simulink model "controlador19"  (R2021a)
settings: Solver=ode23t  StartTime=0.0  StopTime=60  MaxStep=1e-3  RelTol=1e-3
values from neighbouring files (symbols this model uses):
  Ac_2 = [AL-BL*Kes-L*CL+L*DL*Kes, BL*Ki - L*DL*Ki ... (first row only)    [modeloMATEMATICOFINAL.m]
  AL = double(subs(A_par))    [modeloMATEMATICOFINAL.m]
  Bc_2 = [zeros(n,r),L ... (first row only)    [modeloMATEMATICOFINAL.m]
  BL = double(subs(B_par))    [modeloMATEMATICOFINAL.m]
  Blo = 8.18575752786119e-06    (= 8.18575752786e-06)    [modeloMATEMATICOFINAL.m]
  Bmo = 2.02156082362446e-07    (= 2.02156082362e-07)    [modeloMATEMATICOFINAL.m]
  Cc_2 = [-Kes, Ki]    [modeloMATEMATICOFINAL.m]
  CL = double(subs(C_par))    [modeloMATEMATICOFINAL.m]
  Dc_2 = zeros(p,2*r)    [modeloMATEMATICOFINAL.m]
  DL = double(subs(D_par))    [modeloMATEMATICOFINAL.m]
  do = 0.06862-0.021    (= 0.04762)    [modeloMATEMATICOFINAL.m]
  GL = sysd.a    [modeloMATEMATICOFINAL.m]
  go = 9.81    [modeloMATEMATICOFINAL.m]
  HL = sysd.b    [modeloMATEMATICOFINAL.m]
  Jlo = 0.00100697016255642    (= 0.00100697016256)    [modeloMATEMATICOFINAL.m]
  Jmo = 2.08549279330578e-07    (= 2.08549279331e-07)    [modeloMATEMATICOFINAL.m]
  Kes = K(:,1:n)    [modeloMATEMATICOFINAL.m]
  Kest = Kt(:,1:n)    [modeloMATEMATICOFINAL.m]
  Ki = -Kt(:,n+1:end)    [modeloMATEMATICOFINAL.m]
  Kio = 0.00119530882984502    (= 0.00119530882985)    [modeloMATEMATICOFINAL.m]
  Kvo = 0.0035694528924319    (= 0.00356945289243)    [modeloMATEMATICOFINAL.m]
  L = place(GL',CL',pol_obv_d)'    [modeloMATEMATICOFINAL.m]
  Lo = 0.667669785204658    (= 0.667669785205)    [modeloMATEMATICOFINAL.m]
  mo = 0.17244    [modeloMATEMATICOFINAL.m]
  no = 120    [modeloMATEMATICOFINAL.m]
  Ro = 5.15610211779038    (= 5.15610211779)    [modeloMATEMATICOFINAL.m]
  sys_d2 = c2d(sys_c2,Tm)    [modeloMATEMATICOFINAL.m]
  Tm = 0.03    [modeloMATEMATICOFINAL.m]
  Vin0 = Ro*X10    (= 0)    [modeloMATEMATICOFINAL.m]
  X10 = 0    [modeloMATEMATICOFINAL.m]
  X20 = 0    [modeloMATEMATICOFINAL.m]
  X30 = 0    [modeloMATEMATICOFINAL.m]
undefined symbols (not defined in the file or in its folder): magnitude
libraries: simulink x8
settings Model: Creator=hubertdelgado  LastModifiedBy=hubertdelgado

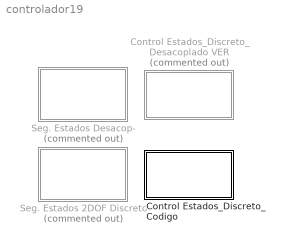
== system controlador19 ==
  Control Estados_Discreto_Codigo : Subsystem
  Control Estados_Discreto_Desacoplado VER : Subsystem  Commented=on
  Seg. Estados 2DOF Discreto : Subsystem  Commented=on
  Seg. Estados Desacop- : Subsystem  Commented=on

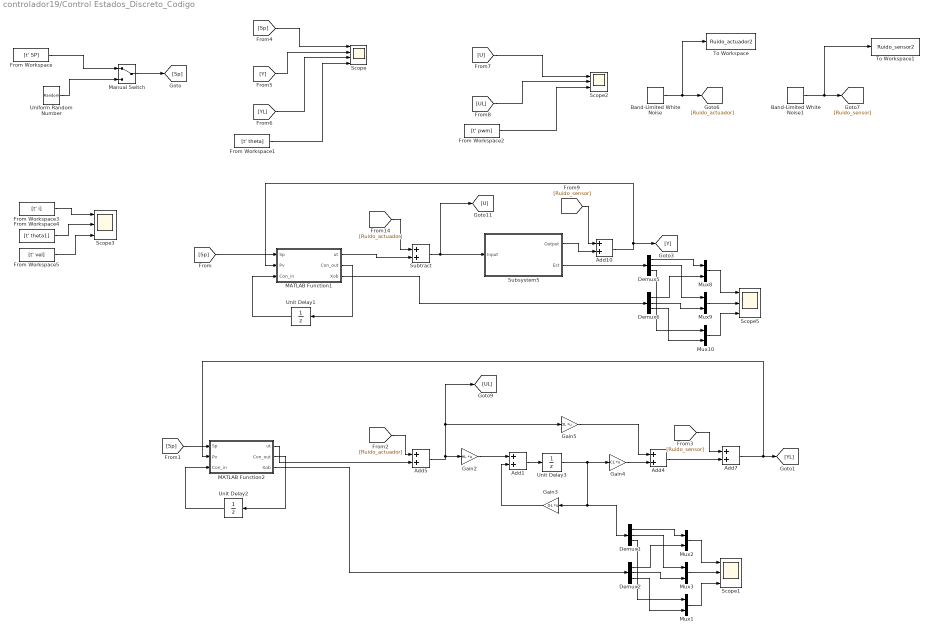
== system controlador19/Control Estados_Discreto_Codigo ==
  Add{1,4..5,7,10} (5 alike) : Sum
  Band-Limited White Noise : simulink/Sources/Band-Limited White Noise  Cov=[1e-8]  Ts=0.001  seed=[23341]
  Band-Limited White Noise1 : simulink/Sources/Band-Limited White Noise  Cov=[1e-8]  Ts=0.001  seed=[23341]
  Demux{1..2,5..6} (4 alike) : Demux  Outputs=3
  From Workspace : FromWorkspace  VariableName=[t' SP]
  From Workspace1 : FromWorkspace  VariableName=[t' theta]
  From Workspace2 : FromWorkspace  VariableName=[t' pwm]
  From Workspace3 : FromWorkspace  VariableName=[t' i]
  From Workspace4 : FromWorkspace  VariableName=[t' theta1]
  From Workspace5 : FromWorkspace  VariableName=[t' vel]
  Gain2 : Gain  Gain=HL  Multiplication=Matrix(K*u)
  Gain3 : Gain  Gain=GL  Multiplication=Matrix(K*u)
  Gain4 : Gain  Gain=CL  Multiplication=Matrix(K*u)
  Gain5 : Gain  Gain=DL  Multiplication=Matrix(K*u)
  MATLAB Function1 : MATLAB Function  TreatAsAtomicUnit=on
  MATLAB Function2 : MATLAB Function  TreatAsAtomicUnit=on
  Manual Switch : ManualSwitch
  Mux{1..3,8..10} (6 alike) : Mux  Inputs=2
  Scope : Scope  NumInputPorts=4
  Scope{1..3,5} (4 alike) : Scope  NumInputPorts=3
  Subsystem5 : Subsystem
  Subtract : Sum
  To Workspace : ToWorkspace  VariableName=Ruido_actuador2  SampleTime=-1
  To Workspace1 : ToWorkspace  VariableName=Ruido_sensor2  SampleTime=-1
  Uniform Random Number : UniformRandomNumber  Minimum=-60*(pi/180)  Maximum=60*(pi/180)  SampleTime=10
  Unit Delay1 : UnitDelay  InitialCondition=zeros(5,1)  SampleTime=Tm  HasFrameUpgradeWarning=on
  Unit Delay2 : UnitDelay  InitialCondition=zeros(5,1)  SampleTime=Tm  HasFrameUpgradeWarning=on
  Unit Delay3 : UnitDelay  SampleTime=Tm  HasFrameUpgradeWarning=on
  wires:
  Add5/1 -> [UL], Gain5/1, Gain2/1
  Add4/1 -> Add7/2
  [Ruido_sensor] -> Add10/1
  [Ruido_actuador] -> Subtract/1
  [Ruido_sensor] -> Add7/1
  Add7/1 -> MATLAB Function2/2(Pv), [YL]
  Gain5/1 -> Add4/1
  Subsystem5/1(Output) -> Add10/2
  MATLAB Function2/1(ut) -> Add5/2
  Subtract/1 -> Subsystem5/1(Input), [U]
  Gain4/1 -> Add4/2
  [Sp] -> MATLAB Function2/1(Sp)
  Band-Limited White Noise/1 -> To Workspace/1, [Ruido_actuador]
  Band-Limited White Noise1/1 -> To Workspace1/1, [Ruido_sensor]
  Gain2/1 -> Add1/1
  Gain3/1 -> Add1/2
  Add1/1 -> Unit Delay3/1
  [Ruido_actuador] -> Add5/1
  MATLAB Function1/2(Con_out) -> Unit Delay1/1
  [Sp] -> MATLAB Function1/1(Sp)
  Unit Delay1/1 -> MATLAB Function1/3(Con_in)
  MATLAB Function1/1(ut) -> Subtract/2
  Add10/1 -> MATLAB Function1/2(Pv), [Y]
  MATLAB Function2/2(Con_out) -> Unit Delay2/1
  Unit Delay2/1 -> MATLAB Function2/3(Con_in)
  Mux8/1 -> Scope5/1
  Mux9/1 -> Scope5/2
  Demux5/3 -> Mux10/1
  Subsystem5/2(Est) -> Demux5/1
  Demux5/1 -> Mux8/1
  Mux10/1 -> Scope5/3
  Demux5/2 -> Mux9/1
  Mux2/1 -> Scope1/1
  Mux3/1 -> Scope1/2
  Demux2/3 -> Mux1/2
  Demux1/3 -> Mux1/1
  Unit Delay3/1 -> Gain4/1, Demux1/1, Gain3/1
  MATLAB Function2/3(Xob) -> Demux2/1
  Demux2/2 -> Mux3/2
  Demux2/1 -> Mux2/2
  Demux1/1 -> Mux2/1
  Mux1/1 -> Scope1/3
  Demux1/2 -> Mux3/1
  From Workspace/1 -> Manual Switch/1
  [Y] -> Scope/2
  From Workspace1/1 -> Scope/4
  Manual Switch/1 -> [Sp]
  [YL] -> Scope/3
  From Workspace2/1 -> Scope2/3
  [UL] -> Scope2/2
  [U] -> Scope2/1
  Uniform Random Number/1 -> Manual Switch/2
  [Sp] -> Scope/1
  From Workspace3/1 -> Scope3/1
  From Workspace4/1 -> Scope3/2
  From Workspace5/1 -> Scope3/3
  MATLAB Function1/3(Xob) -> Demux6/1
  Demux6/1 -> Mux8/2
  Demux6/2 -> Mux9/2
  Demux6/3 -> Mux10/2

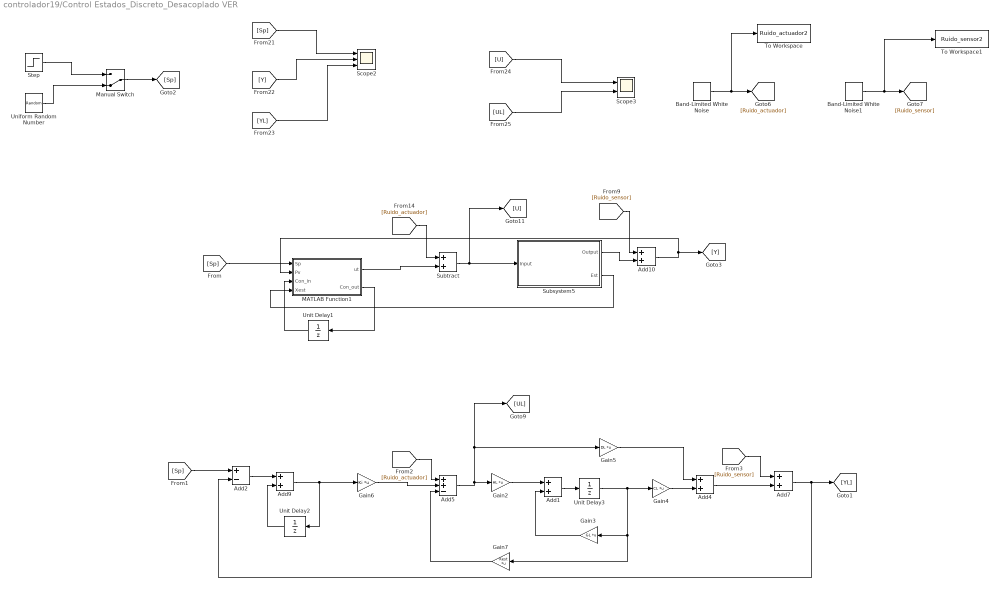
== system controlador19/Control Estados_Discreto_Desacoplado VER ==
  Add{1,4,7,9..10} (5 alike) : Sum
  Add2 : Sum  Inputs=+-
  Add5 : Sum  Inputs=++-
  Band-Limited White Noise : simulink/Sources/Band-Limited White Noise  Cov=[1e-8]  Ts=0.001  seed=[23341]
  Band-Limited White Noise1 : simulink/Sources/Band-Limited White Noise  Cov=[1e-8]  Ts=0.001  seed=[23341]
  Gain2 : Gain  Gain=HL  Multiplication=Matrix(K*u)
  Gain3 : Gain  Gain=GL  Multiplication=Matrix(K*u)
  Gain4 : Gain  Gain=CL  Multiplication=Matrix(K*u)
  Gain5 : Gain  Gain=DL  Multiplication=Matrix(K*u)
  Gain6 : Gain  Gain=Ki  Multiplication=Matrix(K*u)
  Gain7 : Gain  Gain=Kest  Multiplication=Matrix(K*u)
  MATLAB Function1 : MATLAB Function  TreatAsAtomicUnit=on
  Manual Switch : ManualSwitch  CurrentSetting=0
  Scope2 : Scope  NumInputPorts=3
  Scope3 : Scope  NumInputPorts=2
  Step : Step  Time=0  After=30*(pi/180)  SampleTime=0
  Subsystem5 : Subsystem
  Subtract : Sum
  To Workspace : ToWorkspace  VariableName=Ruido_actuador2  SampleTime=-1
  To Workspace1 : ToWorkspace  VariableName=Ruido_sensor2  SampleTime=-1
  Uniform Random Number : UniformRandomNumber  Minimum=-60*(pi/180)  Maximum=60*(pi/180)  SampleTime=10
  Unit Delay1 : UnitDelay  InitialCondition=zeros(2,1)  SampleTime=Tm  HasFrameUpgradeWarning=on
  Unit Delay2 : UnitDelay  SampleTime=Tm  HasFrameUpgradeWarning=on
  Unit Delay3 : UnitDelay  SampleTime=Tm  HasFrameUpgradeWarning=on
  wires:
  [Sp] -> Scope2/1
  Add5/1 -> [UL], Gain5/1, Gain2/1
  Add4/1 -> Add7/2
  [Ruido_sensor] -> Add10/1
  [Ruido_actuador] -> Subtract/1
  [Ruido_sensor] -> Add7/1
  Add7/1 -> Add2/2, [YL]
  Gain5/1 -> Add4/1
  [Y] -> Scope2/2
  Subsystem5/1(Output) -> Add10/2
  [YL] -> Scope2/3
  Subtract/1 -> Subsystem5/1(Input), [U]
  Gain4/1 -> Add4/2
  Band-Limited White Noise/1 -> To Workspace/1, [Ruido_actuador]
  Band-Limited White Noise1/1 -> To Workspace1/1, [Ruido_sensor]
  Manual Switch/1 -> [Sp]
  [UL] -> Scope3/2
  Step/1 -> Manual Switch/1
  [U] -> Scope3/1
  Uniform Random Number/1 -> Manual Switch/2
  Gain2/1 -> Add1/1
  Gain3/1 -> Add1/2
  Add1/1 -> Unit Delay3/1
  [Ruido_actuador] -> Add5/1
  MATLAB Function1/2(Con_out) -> Unit Delay1/1
  [Sp] -> MATLAB Function1/1(Sp)
  Unit Delay1/1 -> MATLAB Function1/3(Con_in)
  MATLAB Function1/1(ut) -> Subtract/2
  Add10/1 -> MATLAB Function1/2(Pv), [Y]
  Unit Delay3/1 -> Gain4/1, Gain7/1, Gain3/1
  Subsystem5/2(Est) -> MATLAB Function1/4(Xest)
  Add9/1 -> Gain6/1, Unit Delay2/1
  Add2/1 -> Add9/1
  Unit Delay2/1 -> Add9/2
  [Sp] -> Add2/1
  Gain6/1 -> Add5/2
  Gain7/1 -> Add5/3

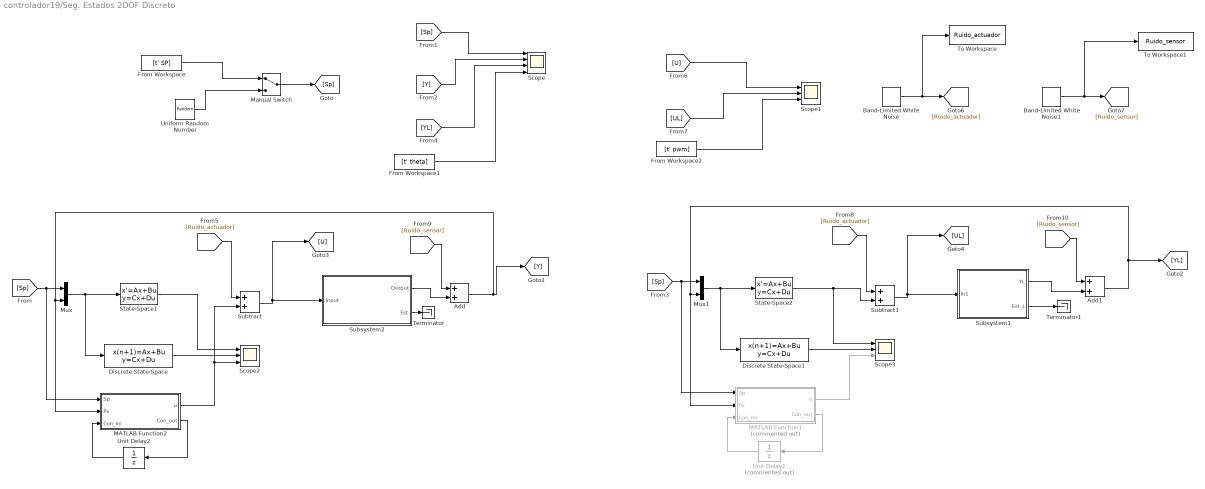
== system controlador19/Seg. Estados 2DOF Discreto ==
  Add : Sum
  Add1 : Sum
  Band-Limited White Noise : simulink/Sources/Band-Limited White Noise  Cov=[1e-8]  Ts=0.001  seed=[23341]
  Band-Limited White Noise1 : simulink/Sources/Band-Limited White Noise  Cov=[1e-8]  Ts=0.001  seed=[23341]
  Discrete State-Space : DiscreteStateSpace  A=sys_d2.a  B=sys_d2.b  C=sys_d2.c  D=sys_d2.d  SampleTime=Tm
  Discrete State-Space1 : DiscreteStateSpace  A=sys_d2.a  B=sys_d2.b  C=sys_d2.c  D=sys_d2.d  SampleTime=Tm
  From Workspace : FromWorkspace  VariableName=[t' SP]
  From Workspace1 : FromWorkspace  VariableName=[t' theta]
  From Workspace2 : FromWorkspace  VariableName=[t' pwm]
  MATLAB Function1 : MATLAB Function  Commented=on  TreatAsAtomicUnit=on
  MATLAB Function2 : MATLAB Function  TreatAsAtomicUnit=on
  Manual Switch : ManualSwitch
  Mux : Mux  Inputs=2
  Mux1 : Mux  Inputs=2
  Scope : Scope  NumInputPorts=4
  Scope1 : Scope  NumInputPorts=3
  Scope2 : Scope  NumInputPorts=3
  Scope3 : Scope  NumInputPorts=3
  State-Space1 : StateSpace  A=Ac_2  B=Bc_2  C=Cc_2  D=Dc_2  InitialCondition=0
  State-Space2 : StateSpace  A=Ac_2  B=Bc_2  C=Cc_2  D=Dc_2  InitialCondition=0
  Subsystem1 : Subsystem
  Subsystem2 : Subsystem
  Subtract : Sum
  Subtract1 : Sum
  Terminator : Terminator
  Terminator1 : Terminator
  To Workspace : ToWorkspace  VariableName=Ruido_actuador  SampleTime=-1
  To Workspace1 : ToWorkspace  VariableName=Ruido_sensor  SampleTime=-1
  Uniform Random Number : UniformRandomNumber  Minimum=-60*(pi/180)  Maximum=60*(pi/180)  SampleTime=10
  Unit Delay1 : UnitDelay  Commented=on  InitialCondition=zeros(8,1)  SampleTime=Tm  HasFrameUpgradeWarning=on
  Unit Delay2 : UnitDelay  InitialCondition=zeros(5,1)  SampleTime=Tm  HasFrameUpgradeWarning=on
  wires:
  [Sp] -> MATLAB Function2/1(Sp), Mux/1
  Band-Limited White Noise/1 -> To Workspace/1, [Ruido_actuador]
  Band-Limited White Noise1/1 -> To Workspace1/1, [Ruido_sensor]
  [UL] -> Scope1/2
  Uniform Random Number/1 -> Manual Switch/2
  [Sp] -> Scope/1
  From Workspace/1 -> Manual Switch/1
  Manual Switch/1 -> [Sp]
  [YL] -> Scope/3
  Subtract/1 -> Subsystem2/1(Input), [U]
  State-Space1/1 -> Scope2/1
  [Ruido_actuador] -> Subtract/1
  Add/1 -> MATLAB Function2/2(Pv), Mux/2, [Y]
  Subsystem2/1(Output) -> Add/2
  [Ruido_sensor] -> Add/1
  Subsystem2/2(Est) -> Terminator/1
  Mux/1 -> Discrete State-Space/1, State-Space1/1
  Discrete State-Space/1 -> Scope2/2
  MATLAB Function2/2(Con_out) -> Unit Delay2/1
  Unit Delay2/1 -> MATLAB Function2/3(Con_ini)
  MATLAB Function2/1(u) -> Subtract/2, Scope2/3
  [Sp] -> MATLAB Function1/1(Sp), Mux1/1
  Subsystem1/2(Est_L) -> Terminator1/1
  MATLAB Function1/1(u) -> Scope3/3
  [Ruido_sensor] -> Add1/1
  Subsystem1/1(YL) -> Add1/2
  Add1/1 -> MATLAB Function1/2(Pv), Mux1/2, [YL]
  Subtract1/1 -> Subsystem1/1(In1), [UL]
  [Ruido_actuador] -> Subtract1/1
  Discrete State-Space1/1 -> Scope3/2
  Unit Delay1/1 -> MATLAB Function1/3(Con_ini)
  Mux1/1 -> Discrete State-Space1/1, State-Space2/1
  State-Space2/1 -> Scope3/1, Subtract1/2
  MATLAB Function1/2(Con_out) -> Unit Delay1/1
  From Workspace1/1 -> Scope/4
  From Workspace2/1 -> Scope1/3
  [Y] -> Scope/2
  [U] -> Scope1/1

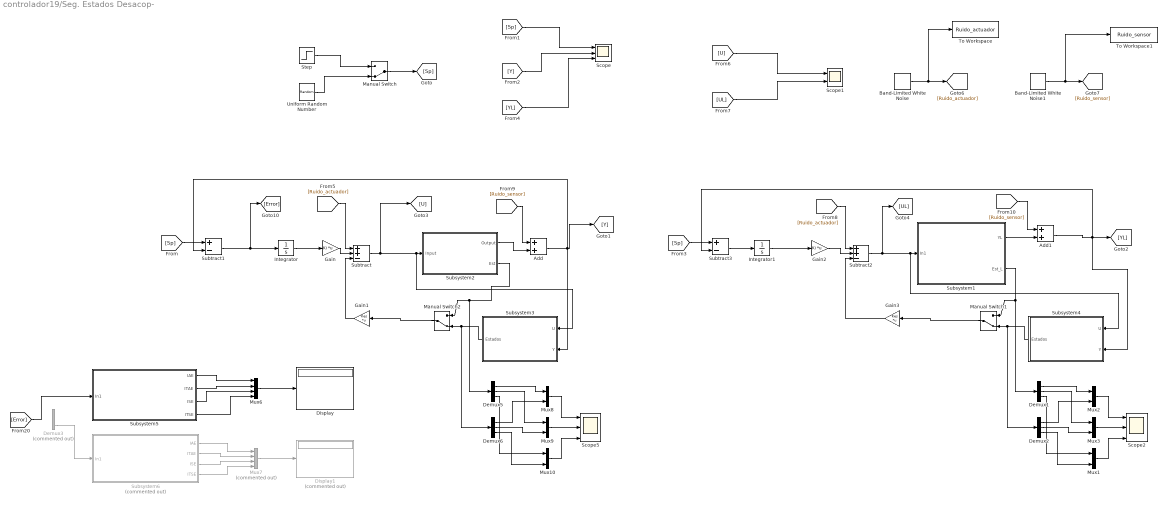
== system controlador19/Seg. Estados Desacop- ==
  Add : Sum
  Add1 : Sum
  Band-Limited White Noise : simulink/Sources/Band-Limited White Noise  Cov=[1e-8]  Ts=0.001  seed=[23341]
  Band-Limited White Noise1 : simulink/Sources/Band-Limited White Noise  Cov=[1e-8]  Ts=0.001  seed=[23341]
  Demux{1..2,5..6} (4 alike) : Demux  Outputs=3
  Demux3 : Demux  Commented=on  Outputs=2
  Display : Display
  Display1 : Display  Commented=on
  Gain : Gain  Gain=Ki  Multiplication=Matrix(K*u)
  Gain1 : Gain  Gain=Kes  Multiplication=Matrix(K*u)
  Gain2 : Gain  Gain=Ki  Multiplication=Matrix(K*u)
  Gain3 : Gain  Gain=Kes  Multiplication=Matrix(K*u)
  Integrator : Integrator
  Integrator1 : Integrator
  Manual Switch : ManualSwitch  CurrentSetting=0
  Manual Switch1 : ManualSwitch  CurrentSetting=0
  Manual Switch2 : ManualSwitch  CurrentSetting=0
  Mux{1..3,8..10} (6 alike) : Mux  Inputs=2
  Mux6 : Mux
  Mux7 : Mux  Commented=on
  Scope : Scope  NumInputPorts=3
  Scope1 : Scope  NumInputPorts=2
  Scope2 : Scope  NumInputPorts=3
  Scope5 : Scope  NumInputPorts=3
  Step : Step  Time=0  After=0  SampleTime=0
  Subsystem1 : Subsystem
  Subsystem2 : Subsystem
  Subsystem3 : Subsystem
  Subsystem4 : Subsystem
  Subsystem5 : Subsystem
  Subsystem6 : Subsystem  Commented=on
  Subtract : Sum  Inputs=++-
  Subtract1 : Sum  Inputs=+-
  Subtract2 : Sum  Inputs=++-
  Subtract3 : Sum  Inputs=+-
  To Workspace : ToWorkspace  VariableName=Ruido_actuador  SampleTime=-1
  To Workspace1 : ToWorkspace  VariableName=Ruido_sensor  SampleTime=-1
  Uniform Random Number : UniformRandomNumber  Minimum=-60*(pi/180)  Maximum=60*(pi/180)  SampleTime=10
  wires:
  [Sp] -> Subtract1/1
  [Sp] -> Subtract3/1
  Integrator/1 -> Gain/1
  Integrator1/1 -> Gain2/1
  Subtract3/1 -> Integrator1/1
  Band-Limited White Noise/1 -> To Workspace/1, [Ruido_actuador]
  Band-Limited White Noise1/1 -> To Workspace1/1, [Ruido_sensor]
  [UL] -> Scope1/2
  Uniform Random Number/1 -> Manual Switch/2
  [Sp] -> Scope/1
  [U] -> Scope1/1
  Step/1 -> Manual Switch/1
  Manual Switch/1 -> [Sp]
  [YL] -> Scope/3
  [Y] -> Scope/2
  Subtract/1 -> Subsystem3/1(U), Subsystem2/1(Input), [U]
  Mux10/1 -> Scope5/3
  Demux6/1 -> Mux8/2
  Demux5/2 -> Mux9/1
  Mux8/1 -> Scope5/1
  Demux6/3 -> Mux10/2
  Demux6/2 -> Mux9/2
  Demux5/3 -> Mux10/1
  Mux9/1 -> Scope5/2
  Subsystem3/1(Estados) -> Demux6/1, Manual Switch2/2
  Subsystem2/2(Est) -> Demux5/1, Manual Switch2/1
  Manual Switch2/1 -> Gain1/1
  Subtract2/1 -> [UL], Subsystem4/1(U), Subsystem1/1(In1)
  Mux1/1 -> Scope2/3
  Demux2/1 -> Mux2/2
  Demux1/2 -> Mux3/1
  Mux2/1 -> Scope2/1
  Demux2/3 -> Mux1/2
  Demux2/2 -> Mux3/2
  Demux1/3 -> Mux1/1
  Mux3/1 -> Scope2/2
  Subsystem4/1(Estados) -> Demux2/1, Manual Switch1/2
  Demux1/1 -> Mux2/1
  Subsystem1/2(Est_L) -> Demux1/1, Manual Switch1/1
  Manual Switch1/1 -> Gain3/1
  Subtract1/1 -> [Error], Integrator/1
  Subsystem5/2(ITAE) -> Mux6/2
  Subsystem5/4(ITSE) -> Mux6/4
  Subsystem5/3(ISE) -> Mux6/3
  Subsystem5/1(IAE) -> Mux6/1
  Mux7/1 -> Display1/1
  Subsystem6/1(IAE) -> Mux7/1
  Subsystem6/4(ITSE) -> Mux7/4
  Mux6/1 -> Display/1
  Demux3/2 -> Subsystem6/1(In1)
  Subsystem6/3(ISE) -> Mux7/3
  Subsystem6/2(ITAE) -> Mux7/2
  [Error] -> Subsystem5/1(In1)
  Gain/1 -> Subtract/2
  Gain1/1 -> Subtract/3
  [Ruido_actuador] -> Subtract/1
  Gain2/1 -> Subtract2/2
  Gain3/1 -> Subtract2/3
  [Ruido_actuador] -> Subtract2/1
  Add/1 -> Subtract1/2, Subsystem3/2(Y), [Y]
  Subsystem2/1(Output) -> Add/2
  [Ruido_sensor] -> Add/1
  Subsystem1/1(YL) -> Add1/2
  Add1/1 -> Subsystem4/2(Y), Subtract3/2, [YL]
  [Ruido_sensor] -> Add1/1
  Demux5/1 -> Mux8/1

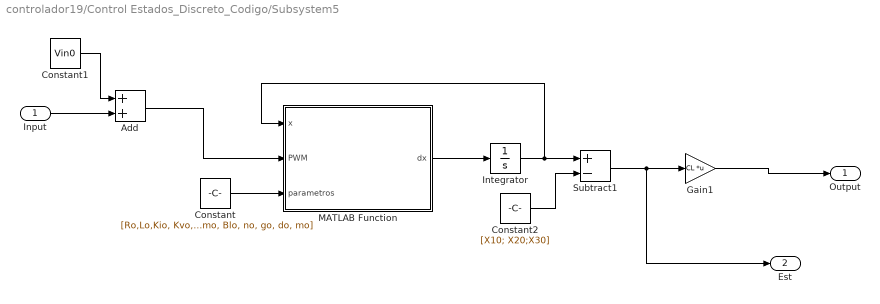
== system controlador19/Control Estados_Discreto_Codigo/Subsystem5 ==
  Input : Inport
  Add : Sum
  Constant : Constant  Value=[Ro,Lo,Kio, Kvo, Jmo, Jlo, Bmo, Blo, no, go, do, mo]
  Constant1 : Constant  Value=Vin0
  Constant2 : Constant  Value=[X10; X20;X30]
  Gain1 : Gain  Gain=CL  Multiplication=Matrix(K*u)
  Integrator : Integrator  InitialCondition=[X10; X20;X30]
  MATLAB Function : MATLAB Function  TreatAsAtomicUnit=on
  Subtract1 : Sum  Inputs=+-
  Output : Outport
  Est : Outport  Port=2
  wires:
  Add/1 -> MATLAB Function/2(PWM)
  Constant2/1 -> Subtract1/2
  Constant1/1 -> Add/1
  Input/1 -> Add/2
  MATLAB Function/1(dx) -> Integrator/1
  Constant/1 -> MATLAB Function/3(parametros)
  Integrator/1 -> Subtract1/1, MATLAB Function/1(x)
  Subtract1/1 -> Est/1, Gain1/1
  Gain1/1 -> Output/1

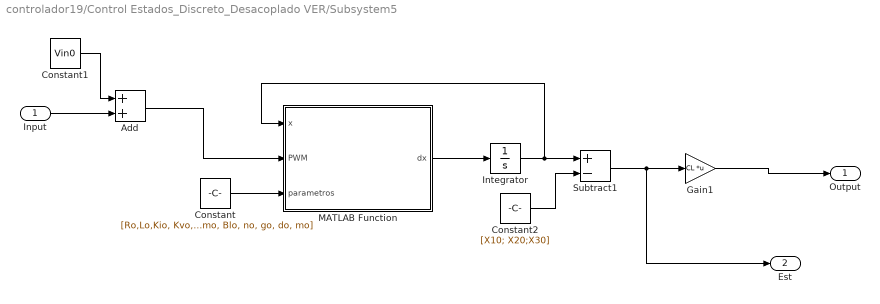
== system controlador19/Control Estados_Discreto_Desacoplado VER/Subsystem5 ==
  Input : Inport
  Add : Sum
  Constant : Constant  Value=[Ro,Lo,Kio, Kvo, Jmo, Jlo, Bmo, Blo, no, go, do, mo]
  Constant1 : Constant  Value=Vin0
  Constant2 : Constant  Value=[X10; X20;X30]
  Gain1 : Gain  Gain=CL  Multiplication=Matrix(K*u)
  Integrator : Integrator  InitialCondition=[X10; X20;X30]
  MATLAB Function : MATLAB Function  TreatAsAtomicUnit=on
  Subtract1 : Sum  Inputs=+-
  Output : Outport
  Est : Outport  Port=2
  wires:
  Add/1 -> MATLAB Function/2(PWM)
  Constant2/1 -> Subtract1/2
  Constant1/1 -> Add/1
  Input/1 -> Add/2
  MATLAB Function/1(dx) -> Integrator/1
  Constant/1 -> MATLAB Function/3(parametros)
  Integrator/1 -> Subtract1/1, MATLAB Function/1(x)
  Subtract1/1 -> Est/1, Gain1/1
  Gain1/1 -> Output/1

== system controlador19/Seg. Estados 2DOF Discreto/Subsystem1 ==
  In1 : Inport
  Add : Sum
  Add1 : Sum
  Gain : Gain  Gain=CL  Multiplication=Matrix(K*u)
  Gain1 : Gain  Gain=AL  Multiplication=Matrix(K*u)
  Gain2 : Gain  Gain=DL  Multiplication=Matrix(K*u)
  Gain3 : Gain  Gain=BL  Multiplication=Matrix(K*u)
  Integrator : Integrator
  YL : Outport
  Est_L : Outport  Port=2
  wires:
  Gain/1 -> Add/2
  Integrator/1 -> Gain/1, Est_L/1, Gain1/1
  Add1/1 -> Integrator/1
  Gain1/1 -> Add1/2
  Gain2/1 -> Add/1
  Gain3/1 -> Add1/1
  Add/1 -> YL/1
  In1/1 -> Gain2/1, Gain3/1

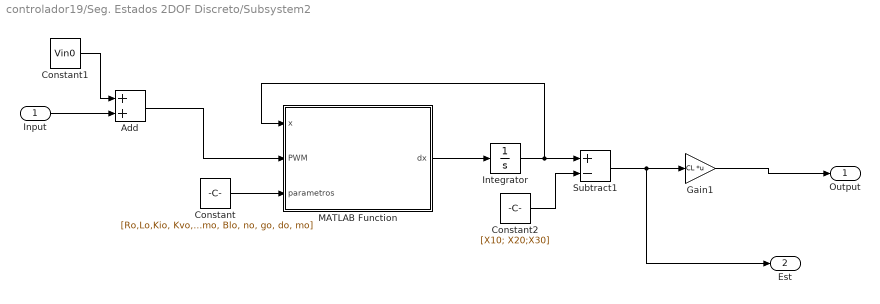
== system controlador19/Seg. Estados 2DOF Discreto/Subsystem2 ==
  Input : Inport
  Add : Sum
  Constant : Constant  Value=[Ro,Lo,Kio, Kvo, Jmo, Jlo, Bmo, Blo, no, go, do, mo]
  Constant1 : Constant  Value=Vin0
  Constant2 : Constant  Value=[X10; X20;X30]
  Gain1 : Gain  Gain=CL  Multiplication=Matrix(K*u)
  Integrator : Integrator  InitialCondition=[X10; X20;X30]
  MATLAB Function : MATLAB Function  TreatAsAtomicUnit=on
  Subtract1 : Sum  Inputs=+-
  Output : Outport
  Est : Outport  Port=2
  wires:
  Add/1 -> MATLAB Function/2(PWM)
  Constant2/1 -> Subtract1/2
  Constant1/1 -> Add/1
  Input/1 -> Add/2
  MATLAB Function/1(dx) -> Integrator/1
  Constant/1 -> MATLAB Function/3(parametros)
  Integrator/1 -> Subtract1/1, MATLAB Function/1(x)
  Subtract1/1 -> Est/1, Gain1/1
  Gain1/1 -> Output/1

== system controlador19/Seg. Estados Desacop-/Subsystem1 ==
  In1 : Inport
  Add : Sum
  Add1 : Sum
  Gain : Gain  Gain=CL  Multiplication=Matrix(K*u)
  Gain1 : Gain  Gain=AL  Multiplication=Matrix(K*u)
  Gain2 : Gain  Gain=DL  Multiplication=Matrix(K*u)
  Gain3 : Gain  Gain=BL  Multiplication=Matrix(K*u)
  Integrator : Integrator
  YL : Outport
  Est_L : Outport  Port=2
  wires:
  Gain/1 -> Add/2
  Integrator/1 -> Gain/1, Est_L/1, Gain1/1
  Add1/1 -> Integrator/1
  Gain1/1 -> Add1/2
  Gain2/1 -> Add/1
  Gain3/1 -> Add1/1
  Add/1 -> YL/1
  In1/1 -> Gain2/1, Gain3/1

== system controlador19/Seg. Estados Desacop-/Subsystem2 ==
  Input : Inport
  Add : Sum
  Constant : Constant  Value=[Ro,Lo,Kio, Kvo, Jmo, Jlo, Bmo, Blo, no, go, do, mo]
  Constant1 : Constant  Value=Vin0
  Constant2 : Constant  Value=[X10; X20;X30]
  Gain1 : Gain  Gain=CL  Multiplication=Matrix(K*u)
  Integrator : Integrator  InitialCondition=[X10; X20;X30]
  MATLAB Function : MATLAB Function  TreatAsAtomicUnit=on
  Subtract1 : Sum  Inputs=+-
  Output : Outport
  Est : Outport  Port=2
  wires:
  Add/1 -> MATLAB Function/2(PWM)
  Constant2/1 -> Subtract1/2
  Constant1/1 -> Add/1
  Input/1 -> Add/2
  MATLAB Function/1(dx) -> Integrator/1
  Constant/1 -> MATLAB Function/3(parametros)
  Integrator/1 -> Subtract1/1, MATLAB Function/1(x)
  Subtract1/1 -> Est/1, Gain1/1
  Gain1/1 -> Output/1

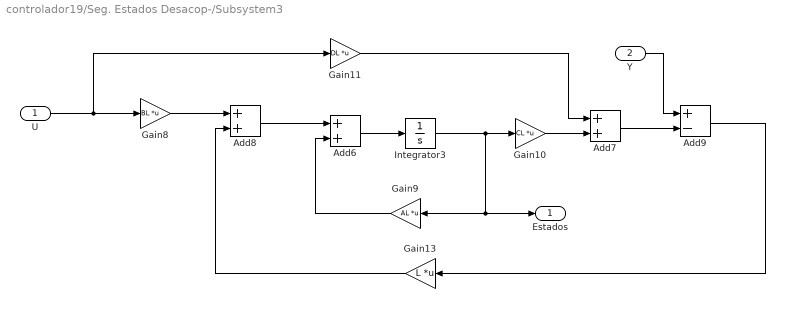
== system controlador19/Seg. Estados Desacop-/Subsystem3 ==
  U : Inport
  Y : Inport  Port=2
  Add6 : Sum
  Add7 : Sum
  Add8 : Sum
  Add9 : Sum  Inputs=+-
  Gain10 : Gain  Gain=CL  Multiplication=Matrix(K*u)
  Gain11 : Gain  Gain=DL  Multiplication=Matrix(K*u)
  Gain13 : Gain  Gain=L  Multiplication=Matrix(K*u)
  Gain8 : Gain  Gain=BL  Multiplication=Matrix(K*u)
  Gain9 : Gain  Gain=AL  Multiplication=Matrix(K*u)
  Integrator3 : Integrator
  Estados : Outport  VectorParamsAs1DForOutWhenUnconnected=off
  wires:
  Gain9/1 -> Add6/2
  Add6/1 -> Integrator3/1
  Integrator3/1 -> Gain9/1, Estados/1, Gain10/1
  Y/1 -> Add9/1
  Add7/1 -> Add9/2
  Add8/1 -> Add6/1
  Add9/1 -> Gain13/1
  Gain13/1 -> Add8/2
  Gain11/1 -> Add7/1
  Gain10/1 -> Add7/2
  Gain8/1 -> Add8/1
  U/1 -> Gain11/1, Gain8/1

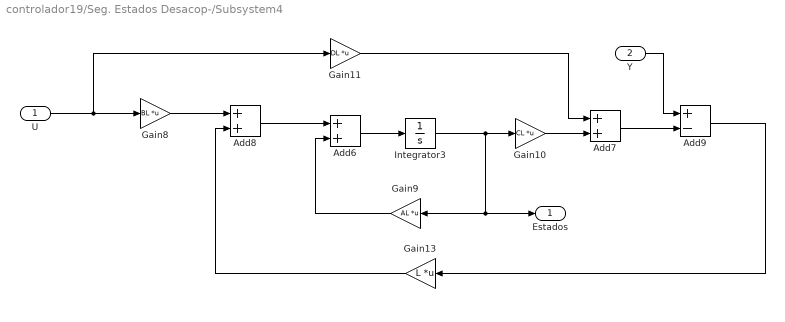
== system controlador19/Seg. Estados Desacop-/Subsystem4 ==
  U : Inport
  Y : Inport  Port=2
  Add6 : Sum
  Add7 : Sum
  Add8 : Sum
  Add9 : Sum  Inputs=+-
  Gain10 : Gain  Gain=CL  Multiplication=Matrix(K*u)
  Gain11 : Gain  Gain=DL  Multiplication=Matrix(K*u)
  Gain13 : Gain  Gain=L  Multiplication=Matrix(K*u)
  Gain8 : Gain  Gain=BL  Multiplication=Matrix(K*u)
  Gain9 : Gain  Gain=AL  Multiplication=Matrix(K*u)
  Integrator3 : Integrator
  Estados : Outport  VectorParamsAs1DForOutWhenUnconnected=off
  wires:
  Gain9/1 -> Add6/2
  Add6/1 -> Integrator3/1
  Integrator3/1 -> Gain9/1, Estados/1, Gain10/1
  Y/1 -> Add9/1
  Add7/1 -> Add9/2
  Add8/1 -> Add6/1
  Add9/1 -> Gain13/1
  Gain13/1 -> Add8/2
  Gain11/1 -> Add7/1
  Gain10/1 -> Add7/2
  Gain8/1 -> Add8/1
  U/1 -> Gain11/1, Gain8/1

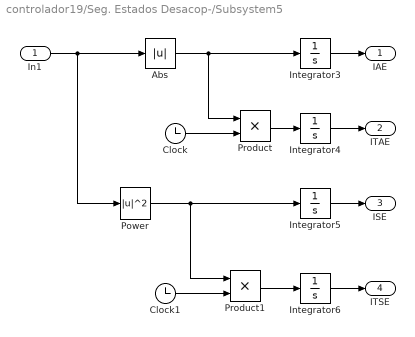
== system controlador19/Seg. Estados Desacop-/Subsystem5 ==
  In1 : Inport
  Abs : Abs
  Clock : Clock
  Clock1 : Clock
  Integrator{3..6} (4 alike) : Integrator
  Power : Math  Operator=magnitude^2  SignedPower=on  SaturateOnIntegerOverflow=on
  Product : Product
  Product1 : Product
  IAE : Outport  VectorParamsAs1DForOutWhenUnconnected=off
  ITAE : Outport  Port=2  VectorParamsAs1DForOutWhenUnconnected=off
  ISE : Outport  Port=3  VectorParamsAs1DForOutWhenUnconnected=off
  ITSE : Outport  Port=4  VectorParamsAs1DForOutWhenUnconnected=off
  wires:
  Clock/1 -> Product/2
  Power/1 -> Integrator5/1, Product1/1
  Product1/1 -> Integrator6/1
  Abs/1 -> Product/1, Integrator3/1
  Clock1/1 -> Product1/2
  Product/1 -> Integrator4/1
  Integrator3/1 -> IAE/1
  Integrator6/1 -> ITSE/1
  Integrator4/1 -> ITAE/1
  In1/1 -> Power/1, Abs/1
  Integrator5/1 -> ISE/1

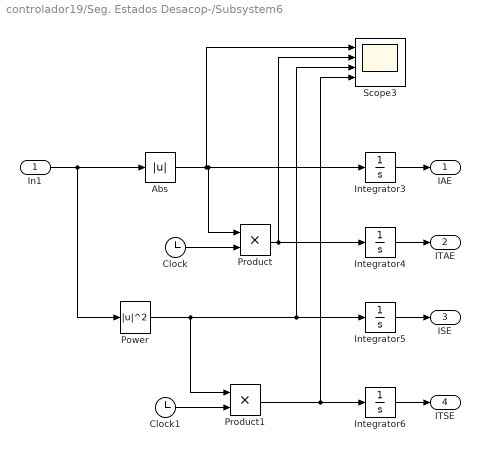
== system controlador19/Seg. Estados Desacop-/Subsystem6 ==
  In1 : Inport
  Abs : Abs
  Clock : Clock
  Clock1 : Clock
  Integrator{3..6} (4 alike) : Integrator
  Power : Math  Operator=magnitude^2  SignedPower=on  SaturateOnIntegerOverflow=on
  Product : Product
  Product1 : Product
  Scope3 : Scope  NumInputPorts=4
  IAE : Outport  VectorParamsAs1DForOutWhenUnconnected=off
  ITAE : Outport  Port=2  VectorParamsAs1DForOutWhenUnconnected=off
  ISE : Outport  Port=3  VectorParamsAs1DForOutWhenUnconnected=off
  ITSE : Outport  Port=4  VectorParamsAs1DForOutWhenUnconnected=off
  wires:
  Integrator5/1 -> ISE/1
  In1/1 -> Abs/1, Power/1
  Integrator4/1 -> ITAE/1
  Integrator6/1 -> ITSE/1
  Integrator3/1 -> IAE/1
  Product/1 -> Scope3/2, Integrator4/1
  Clock1/1 -> Product1/2
  Abs/1 -> Scope3/1, Integrator3/1, Product/1
  Product1/1 -> Scope3/4, Integrator6/1
  Power/1 -> Product1/1, Scope3/3, Integrator5/1
  Clock/1 -> Product/2

== matlab function controlador19/Control Estados_Discreto_Codigo/Subsystem5/MATLAB Function ==
  data: x input; PWM input; dx output; parametros input
function dx = fcn(x,PWM,parametros)

%ESTADOS
x1 = x(1);
x2 = x(2);
x3 = x(3);

%Parametros
R = parametros(1);
L = parametros(2);
Ki = parametros(3);
Kv = parametros(4);
Jm = parametros(5);
Jl = parametros(6);
Bm = parametros(7);
Bl = parametros(8);
n = parametros(9);
g = parametros(10);
d = parametros(11);
m = parametros(12);

%EXPRESIONES
% Jt = Jm*n^2 +Jl;
% f1 = (1/L)*(((7*PWM)/100) - R*x1 - Kv*x2*n);
% f2 = (1/Jt)*(Ki*x1*n - (Bm*n^2 + Bl)*x2 - m*g*d*sin(x3));
% f3 = x2;

% MODELO 2 ESTADOS I TL WL  SALIDA TL WL
f1 = (((7*PWM)/100)-Kv*x3*n-R*x1)/(L); %di/dt
f2 = x3; %d0l/dt = Wl
f3 = ((Ki*x1*n)-x3*(Bm*n^2+Bl)-(m*g*d*sin(x2)))/(Jl+Jm*n^2);  %dwl/dt 

dx = [f1; f2; f3];

== matlab function controlador19/Control Estados_Discreto_Codigo/MATLAB Function2 ==
  data: Sp input; ut output; Pv input; Con_in input; Con_out output; Xob output
function [ut,Con_out,Xob] = fcn(Sp,Pv,Con_in)
Vk_1 = Con_in(1); % Número de integradores
Xk_1 = Con_in(2:4); % Estados planta
Du = Con_in(5); % Actuadores

u1max = 100;
u1min = -100;

Ka = zeros(1,1);  %(r,p)

GL = [0.784437384092603,0.00531930682271875,-0.0168735214917902;0.0147638228309042,0.991053908598640,0.0294892447225049;0.940790474483479,-0.592389086150106,0.960114981651867];
HL = [0.00279792290617123;1.58234863317437e-05;0.00154787234807474];
CL = [0,1,0];
Ki = [2.208069660656375];
Kest = [106.389627162668,4.54202985096176,22.5481367796194];
%L = [0.0908370092518715;0.122492624265940;-1.34405909478463]; %Luenberger
L = [1.97870165160901e-06;4.44347573756390e-05;-2.44210589797653e-05]; %KALMAN


en = Sp-Pv;
Vk = en + Vk_1 - Ka*Du;
u = Ki*Vk - Kest*Xk_1;
Xob = (GL-L*CL)*Xk_1 + HL*u + L*Pv;

u1s = u(1);

if u(1)>=u1max
    u1s = u1max;
end
if u(1)<=u1min
    u1s = u1min;
end



%% Salida
ut = u1s;
Dunew = u - ut;
Con_out = [Vk; Xob; Dunew];

== matlab function controlador19/Control Estados_Discreto_Desacoplado VER/MATLAB Function1 ==
  data: Sp input; ut output; Pv input; Con_in input; Con_out output; Xest input
function [ut,Con_out] = fcn(Sp,Pv,Con_in, Xest)
Vk_1 = Con_in(1); % Número de integradores
Du = Con_in(2); % Actuadores

u1max = 100;
u1min = -100;

Ka = zeros(1,1);  %(r,p)

Ki = [2.208069660656375];
Kest = [106.389627162668,4.54202985096176,22.5481367796194];


en = Sp-Pv;
Vk = en + Vk_1 - Ka*Du;
u = Ki*Vk - Kest*Xest;

u1s = u(1);

if u(1)>=u1max
    u1s = u1max;
end
if u(1)<=u1min
    u1s = u1min;
end



%% Salida
ut = u1s;
Dunew = u - ut;
Con_out = [Vk; Dunew];

== matlab function controlador19/Seg. Estados Desacop-/Subsystem2/MATLAB Function ==
  data: x input; PWM input; dx output; parametros input
function dx = fcn(x,PWM,parametros)

%ESTADOS
x1 = x(1);
x2 = x(2);
x3 = x(3);

%Parametros
R = parametros(1);
L = parametros(2);
Ki = parametros(3);
Kv = parametros(4);
Jm = parametros(5);
Jl = parametros(6);
Bm = parametros(7);
Bl = parametros(8);
n = parametros(9);
g = parametros(10);
d = parametros(11);
m = parametros(12);

%EXPRESIONES
% Jt = Jm*n^2 +Jl;
% f1 = (1/L)*(((7*PWM)/100) - R*x1 - Kv*x2*n);
% f2 = (1/Jt)*(Ki*x1*n - (Bm*n^2 + Bl)*x2 - m*g*d*sin(x3));
% f3 = x2;

% MODELO 2 ESTADOS I TL WL  SALIDA TL WL
f1 = (((7*PWM)/100)-Kv*x3*n-R*x1)/(L); %di/dt
f2 = x3; %d0l/dt = Wl
f3 = ((Ki*x1*n)-x3*(Bm*n^2+Bl)-(m*g*d*sin(x2)))/(Jl+Jm*n^2);  %dwl/dt 

dx = [f1; f2; f3];

== matlab function controlador19/Seg. Estados 2DOF Discreto/Subsystem2/MATLAB Function ==
  data: x input; PWM input; dx output; parametros input
function dx = fcn(x,PWM,parametros)

%ESTADOS
x1 = x(1);
x2 = x(2);
x3 = x(3);

%Parametros
R = parametros(1);
L = parametros(2);
Ki = parametros(3);
Kv = parametros(4);
Jm = parametros(5);
Jl = parametros(6);
Bm = parametros(7);
Bl = parametros(8);
n = parametros(9);
g = parametros(10);
d = parametros(11);
m = parametros(12);

%EXPRESIONES
% Jt = Jm*n^2 +Jl;
% f1 = (1/L)*(((7*PWM)/100) - R*x1 - Kv*x2*n);
% f2 = (1/Jt)*(Ki*x1*n - (Bm*n^2 + Bl)*x2 - m*g*d*sin(x3));
% f3 = x2;

% MODELO 2 ESTADOS I TL WL  SALIDA TL WL
f1 = (((7*PWM)/100)-Kv*x3*n-R*x1)/(L); %di/dt
f2 = x3; %d0l/dt = Wl
f3 = ((Ki*x1*n)-x3*(Bm*n^2+Bl)-(m*g*d*sin(x2)))/(Jl+Jm*n^2);  %dwl/dt 

dx = [f1; f2; f3];

== matlab function controlador19/Seg. Estados 2DOF Discreto/MATLAB Function2 ==
  data: Sp input; u output; Pv input; Con_ini input; Con_out output
function [u,Con_out] = fcn(Sp,Pv,Con_ini)
Gc = [0.523966818008876,0.0782855124325541,-0.100820826191194,0.105348989718112;0.0132088738475635,0.991367484590253,0.0289530105661962,0.000651705484506732;0.791279836062320,-0.555522722213387,0.909698456385056,0.0619332601210404;0,0,0,1];
Hc = [0.00174756461598906,-0.00174430609133644;5.03642823964450e-06,3.97073674635666e-05;0.000651713016402831,-0.000663568108338496;0.0300000000000000,-0.0300000000000000];
Cc = [-102.796775094684,18.8434497806392,-37.6657368965831,44.7213595499957];
Dc = [0	0];

u1max = 100;
u1min = -100;

Ka = zeros(4,1);

xk = Con_ini(1:4);  %n+r
Du = Con_ini(5:5);  %p

u = Cc*xk + Dc*[Sp;Pv];
xk_1 = Gc*xk + Hc*[Sp;Pv] - Ka*Du;

% Hsp = [0.000536712016934462,0.000277774040110453;0.00110188262899529,-0.000214997449972678;5.70600160926339e-05,0.000178431372314633;0.000111261745162715,-0.000748573895925450;0.0600000000000000,0;0,0.0600000000000000];
% Hpv = [0.528743127428489,-0.0440381830752178;0.441160175174069,0.0425524022491926;-0.00772595368821204,0.204727393044363;-0.0185719938075179,0.0357506408044768;-0.0600000000000000,0;0,-0.0600000000000000];
% u = Cc*xk;
% xk_1 = Gc*xk + Hsp*Sp + Hpv*Pv - Ka*Du;

u1s = u(1);

if u(1)>=u1max
    u1s = u1max;
end
if u(1)<=u1min
    u1s = u1min;
end



%% Salida
ut = u1s;
Dunew = u - ut;
Con_out = [xk_1; Dunew];

== matlab function controlador19/Seg. Estados 2DOF Discreto/MATLAB Function1 ==
  data: Sp input; u output; Pv input; Con_ini input; Con_out output
function [u,Con_out] = fcn(Sp,Pv,Con_ini)
Gc = [0.883560462392427	-4.13249708388486e-12	-0.00487572121212935	0.135443000110772	-0.00479641932613010
-0.000588434369415533	0.644036421083143	0.00829798816152157	-4.57027036271401e-05	0.00866807794337489
-0.00487572121200123	1.30651084000254e-14	0.577392998520158	-0.000392434304393785	1.35422668727884
0	0	0	1	0
0	0	0	0	1];
Hc = [0.00138236824312267	-3.37592528540001e-05	0.00971261372273124	0.00632660435715394
-3.16147125121532e-07	6.26926980241918e-05	0.000624297068749436	-0.0109217038882698
-2.76212064284266e-06	0.0147757234577708	0.00518371001609480	0.00771884768968612
0.0200000000000000	0	-0.0200000000000000	0
0	0.0200000000000000	0	-0.0200000000000000];
Cc = [2.60000000006463	3.87499999993181	-0.750000000024670	1.79999999984347	9.96447369061571e-11
-4.30872282297656e-11	-2.25000000000000	0.499999999999999	1.04354552776798e-10	1.64313007644523e-14
-2.80000000007810	-1.93749999996589	-11.1249999999877	-0.899999999768644	43.9999999999502];
Dc = [0	0	0	0
0	0	0	0
0	0	0	0];

u1max = 10;
u1min = -10;
u2max = 10;
u2min = -10;
u3max = 10;
u3min = -10;

Ka = zeros(5,3);

xk = Con_ini(1:5);  %n+r
Du = Con_ini(6:8);  %p

u = Cc*xk + Dc*[Sp;Pv];
xk_1 = Gc*xk + Hc*[Sp;Pv] - Ka*Du;

% Hsp = [0.000536712016934462,0.000277774040110453;0.00110188262899529,-0.000214997449972678;5.70600160926339e-05,0.000178431372314633;0.000111261745162715,-0.000748573895925450;0.0600000000000000,0;0,0.0600000000000000];
% Hpv = [0.528743127428489,-0.0440381830752178;0.441160175174069,0.0425524022491926;-0.00772595368821204,0.204727393044363;-0.0185719938075179,0.0357506408044768;-0.0600000000000000,0;0,-0.0600000000000000];
% u = Cc*xk;
% xk_1 = Gc*xk + Hsp*Sp + Hpv*Pv - Ka*Du;

u1s = u(1);
u2s = u(2);
u3s = u(3);

if u(1)>=u1max
    u1s = u1max;
end
if u(1)<=u1min
    u1s = u1min;
end

if u(2)>=u2max
    u2s = u2max;
end
if u(2)<=u2min
    u2s = u2min;
end

if u(3)>=u3max
    u3s = u3max;
end
if u(3)<=u3min
    u3s = u3min;
end

%% Salida
ut = [u1s;u2s;u3s];
Dunew = u - ut;
Con_out = [xk_1; Dunew];

== matlab function controlador19/Control Estados_Discreto_Desacoplado VER/Subsystem5/MATLAB Function ==
  data: x input; PWM input; dx output; parametros input
function dx = fcn(x,PWM,parametros)

%ESTADOS
x1 = x(1);
x2 = x(2);
x3 = x(3);

%Parametros
R = parametros(1);
L = parametros(2);
Ki = parametros(3);
Kv = parametros(4);
Jm = parametros(5);
Jl = parametros(6);
Bm = parametros(7);
Bl = parametros(8);
n = parametros(9);
g = parametros(10);
d = parametros(11);
m = parametros(12);

%EXPRESIONES
% Jt = Jm*n^2 +Jl;
% f1 = (1/L)*(((7*PWM)/100) - R*x1 - Kv*x2*n);
% f2 = (1/Jt)*(Ki*x1*n - (Bm*n^2 + Bl)*x2 - m*g*d*sin(x3));
% f3 = x2;

% MODELO 2 ESTADOS I TL WL  SALIDA TL WL
f1 = (((7*PWM)/100)-Kv*x3*n-R*x1)/(L); %di/dt
f2 = x3; %d0l/dt = Wl
f3 = ((Ki*x1*n)-x3*(Bm*n^2+Bl)-(m*g*d*sin(x2)))/(Jl+Jm*n^2);  %dwl/dt 

dx = [f1; f2; f3];

== matlab function controlador19/Control Estados_Discreto_Codigo/MATLAB Function1 ==
  data: Sp input; ut output; Pv input; Con_in input; Con_out output; Xob output
function [ut,Con_out,Xob] = fcn(Sp,Pv,Con_in)
Vk_1 = Con_in(1); % Número de integradores
Xk_1 = Con_in(2:4); % Estados planta
Du = Con_in(5); % Actuadores

u1max = 100;
u1min = -100;

Ka = zeros(1,1);  %(r,p)

GL = [0.784437384092603,0.00531930682271875,-0.0168735214917902;0.0147638228309042,0.991053908598640,0.0294892447225049;0.940790474483479,-0.592389086150106,0.960114981651867];
HL = [0.00279792290617123;1.58234863317437e-05;0.00154787234807474];
CL = [0,1,0];
Ki = [2.208069660656375];
Kest = [106.389627162668,4.54202985096176,22.5481367796194];
%L = [0.0908370092518715;0.122492624265940;-1.34405909478463]; %Luenberger
L = [1.97870165160901e-06;4.44347573756390e-05;-2.44210589797653e-05]; %KALMAN


en = Sp-Pv;
Vk = en + Vk_1 - Ka*Du;
u = Ki*Vk - Kest*Xk_1;
Xob = (GL-L*CL)*Xk_1 + HL*u + L*Pv;

u1s = u(1);

if u(1)>=u1max
    u1s = u1max;
end
if u(1)<=u1min
    u1s = u1min;
end



%% Salida
ut = u1s;
Dunew = u - ut;
Con_out = [Vk; Xob; Dunew];
